simulink model "fixed_load_capacitor_bank"  (R2023b)
settings: Solver=VariableStepAuto  StartTime=0.0  StopTime=1  RelTol=1e-3
libraries: spsRMSLib x3, spsSeriesRLCLoadLib x2, eePowerMeasurement x2, spsVoltageMeasurementLib x2, spsCurrentMeasurementLib x1, spsSeriesRLCBranchLib x1, spsACVoltageSourceLib x1, sps_lib x1
settings Model: Creator=ASUS  LastModifiedBy=ASUS

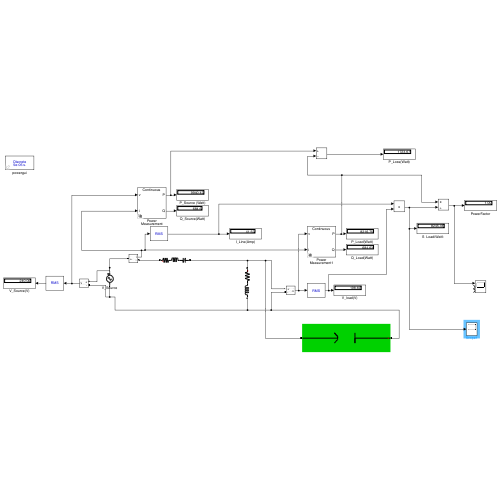
[thumbnail: Simulink's stored preview of the top-level diagram]
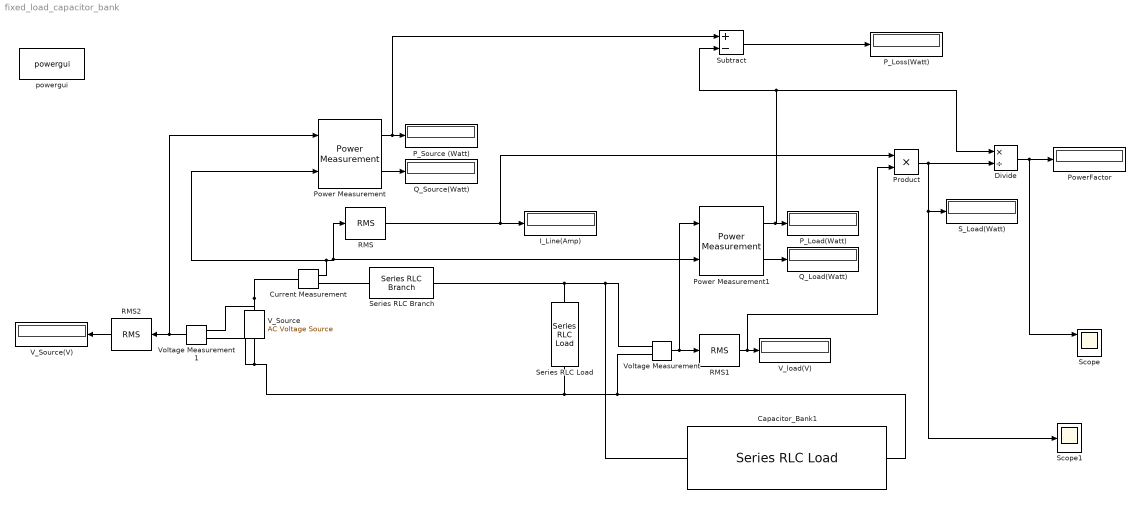
== system fixed_load_capacitor_bank ==
  Capacitor_Bank1 : spsSeriesRLCLoadLib/Series RLC Load  LConnTagsString=a  RConnTagsString=__new0  NominalVoltage=120  NominalFrequency=60  ActivePower=0  InductivePower=0  CapacitivePower=2000  Setx0=off  InitialVoltage=0  SetiL0=off  InitialCurrent=0  Measurements=None  LoadType=constant Z
  Current Measurement : spsCurrentMeasurementLib/Current Measurement  PhasorSimulation=off  OutputType=Complex  PSBequivalent=0
  Divide : Product  Inputs=*/
  I_Line(Amp) : Display
  P_Load(Watt) : Display
      settings: Format=bank
  P_Loss(Watt) : Display
      settings: Format=bank
  P_Source (Watt) : Display
      settings: Format=bank
  Power Measurement : eePowerMeasurement/Power Measurement  LabelModeActiveChoice=Continuous  F=60  K=[1]  Ts=0
  Power Measurement1 : eePowerMeasurement/Power Measurement  LabelModeActiveChoice=Continuous  F=60  K=[1]  Ts=0
  PowerFactor : Display
      settings: Format=bank
  Product : Product
  Q_Load(Watt) : Display
      settings: Format=bank
  Q_Source(Watt) : Display
  RMS : spsRMSLib/RMS  TrueRMS=on  Freq=60  RMSInit=120  Ts=0
  RMS1 : spsRMSLib/RMS  TrueRMS=on  Freq=60  RMSInit=120  Ts=0
  RMS2 : spsRMSLib/RMS  TrueRMS=on  Freq=60  RMSInit=120  Ts=0
  S_Load(Watt) : Display
      settings: Format=bank
  Scope : Scope  NumInputPorts=3
  Scope1 : Scope
  Series RLC Branch : spsSeriesRLCBranchLib/Series RLC Branch  LConnTagsString=__new0  RConnTagsString=__new0  BranchType=RLC  Resistance=1  Inductance=0  SetiL0=off  InitialCurrent=0  Capacitance=0  Setx0=off  InitialVoltage=0  Measurements=None
  Series RLC Load : spsSeriesRLCLoadLib/Series RLC Load  LConnTagsString=a  RConnTagsString=__new0  NominalVoltage=120  NominalFrequency=60  ActivePower=3000  InductivePower=2250  CapacitivePower=0  Setx0=off  InitialVoltage=0  SetiL0=off  InitialCurrent=0  Measurements=None  LoadType=constant Z
  Subtract : Sum  Inputs=+-
  V_Source : spsACVoltageSourceLib/AC Voltage Source  Amplitude=240*sqrt(2)  Phase=0  Frequency=60  SampleTime=0  Measurements=None  BusType=swing  Pref=10e3  Qref=0  Qmin=-inf  Qmax=+inf
  V_Source(V) : Display
      settings: Format=bank
  V_load(V) : Display
      settings: Format=bank
  Voltage Measurement : spsVoltageMeasurementLib/Voltage Measurement  PhasorSimulation=off  OutputType=Complex  PSBequivalent=0
  Voltage Measurement1 : spsVoltageMeasurementLib/Voltage Measurement  PhasorSimulation=off  OutputType=Complex  PSBequivalent=0
  powergui : sps_lib/powergui  Priority=1  SimulationMode=Discrete  SampleTime=50e-6  frequency=60  Iterations=50  frequencyindice=60  Pbase=100e6  ErrMax=1e-4  UnitsV=kV  UnitsW=MW  buscounter=0  FunctionMessages=off  echomessages=off  EnableUseOfTLC=off  CurrentSourceSwitches=off  DisableSnubberDevices=off  DisableRonSwitches=off  DisableVfSwitches=off  DisplayEquations=off  AutomaticDiscreteSolvers=off  SolverType=Tustin/Backward Euler (TBE)  Interpol=off  ExternalGateDelay=off  methode=off  Ts=100  x0status=blocks  SPID=on  SwTol=0  HookPort=off  NonlinearTolerance=1e-4  nMaxIteration=100  ContinueOnMaxIteration=off  RestoreLinks=warning  ResistiveCurrentMeasurement=off  Frange=[0:2:500]  Ylog=off  Xlog=on  ShowGrid=off  save=off  variable=ZData  structure=0  ZoomFFT=off  StartTime=0.0  cycles=1  DisplayStyle=1  fundamental=60  FreqAxis=off  MaxFrequency=1000  frequencyindicesteady=1  RmsSteady=1  display=off
  wires:
  Current Measurement/1 -> Power Measurement1/2, RMS/1, Power Measurement/2
  RMS/1 -> Product/1, I_Line(Amp)/1
  Voltage Measurement/1 -> Power Measurement1/1, RMS1/1
  RMS1/1 -> Product/2, V_load(V)/1
  RMS2/1 -> V_Source(V)/1
  Voltage Measurement1/1 -> Power Measurement/1, RMS2/1
  Power Measurement/2 -> Q_Source(Watt)/1
  Power Measurement/1 -> Subtract/1, P_Source (Watt)/1
  Power Measurement1/1 -> Subtract/2, Divide/1, P_Load(Watt)/1
  Power Measurement1/2 -> Q_Load(Watt)/1
  Subtract/1 -> P_Loss(Watt)/1
  Product/1 -> Scope1/1, S_Load(Watt)/1, Divide/2
  Divide/1 -> Scope/1, PowerFactor/1
  connections:
  V_Source/RConn1 -- Current Measurement/LConn1 -- Voltage Measurement1/LConn1
  Series RLC Branch/RConn1 -- Series RLC Load/LConn1 -- Capacitor_Bank1/RConn1 -- Voltage Measurement/LConn1
  V_Source/LConn1 -- Voltage Measurement1/LConn2 -- Series RLC Load/RConn1 -- Capacitor_Bank1/LConn1 -- Voltage Measurement/LConn2
  Series RLC Branch/LConn1 -- Current Measurement/RConn1
